simulink model "motor_error"  (R2018b)
settings: Solver=FixedStepAuto  StartTime=0.0  StopTime=10.0  FixedStep=0.001  RelTol=1e-3
settings Model: Creator=chengqian  LastModifiedBy=chengqian

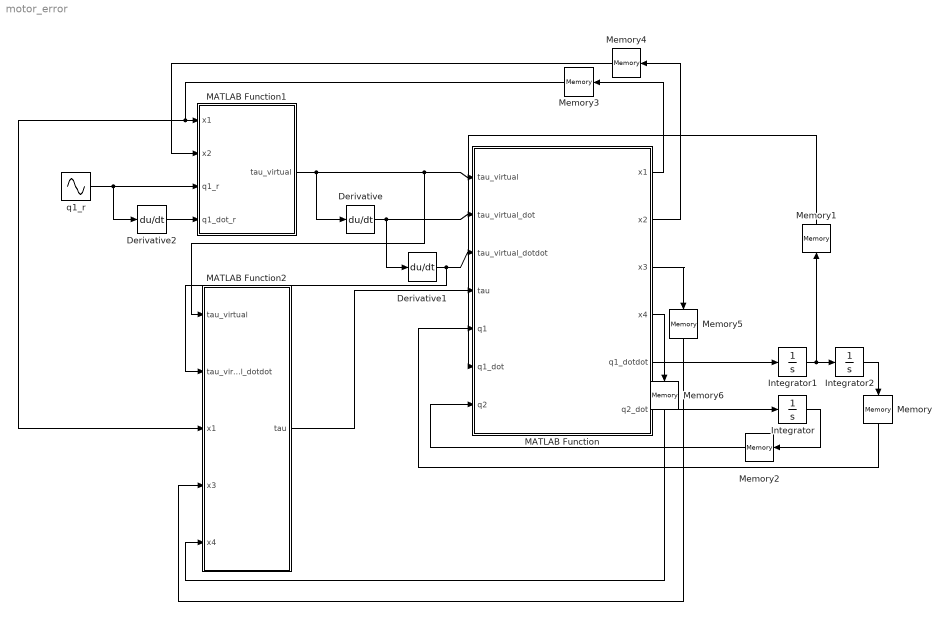
== system motor_error ==
  Derivative : Derivative
  Derivative1 : Derivative
  Derivative2 : Derivative
  Integrator : Integrator
  Integrator1 : Integrator
  Integrator2 : Integrator
  MATLAB Function : MATLAB Function  TreatAsAtomicUnit=on
  MATLAB Function1 : MATLAB Function  TreatAsAtomicUnit=on
  MATLAB Function2 : MATLAB Function  TreatAsAtomicUnit=on
  Memory{,1..6} (7 alike) : Memory
  q1_r : Sin  SampleTime=0
  wires:
  MATLAB Function1/1(tau_virtual) -> Derivative/1, MATLAB Function2/1(tau_virtual), MATLAB Function/1(tau_virtual)
  Derivative/1 -> Derivative1/1, MATLAB Function/2(tau_virtual_dot)
  Derivative1/1 -> MATLAB Function2/2(tau_virtual_dotdot), MATLAB Function/3(tau_virtual_dotdot)
  MATLAB Function/6(q2_dot) -> Integrator/1
  Integrator/1 -> Memory2/1
  MATLAB Function/5(q1_dotdot) -> Integrator1/1
  Integrator2/1 -> Memory/1
  MATLAB Function/1(x1) -> Memory3/1
  MATLAB Function/2(x2) -> Memory4/1
  q1_r/1 -> Derivative2/1, MATLAB Function1/3(q1_r)
  Derivative2/1 -> MATLAB Function1/4(q1_dot_r)
  MATLAB Function2/1(tau) -> MATLAB Function/4(tau)
  MATLAB Function/4(x4) -> Memory6/1
  MATLAB Function/3(x3) -> Memory5/1
  Integrator1/1 -> Integrator2/1, Memory1/1
  Memory/1 -> MATLAB Function/5(q1)
  Memory1/1 -> MATLAB Function/6(q1_dot)
  Memory2/1 -> MATLAB Function/7(q2)
  Memory3/1 -> MATLAB Function2/3(x1), MATLAB Function1/1(x1)
  Memory4/1 -> MATLAB Function1/2(x2)
  Memory5/1 -> MATLAB Function2/4(x3)
  Memory6/1 -> MATLAB Function2/5(x4)

== matlab function motor_error/MATLAB Function1 ==
  data: x1 input; tau_virtual output; x2 input; q1_r input; q1_dot_r input
function tau_virtual = fcn(x1,x2,q1_r,q1_dot_r)

T = 10;
J = 0.0101;
M = 0.0320;
K = 4000;

beta1 = 2; beta2 = 2;
alpha1 = 10; alpha2 = 10;
Kp1 = 100; Kd1 =20;

rol1 = norm((-T - K*x1 + M*x2));
e1 = q1_r - x1;
e2 = q1_dot_r - x2;
tau_virtual = (1/K)*((-alpha1*rol1^2-beta1)*(x1+x2) + (-Kp1*e1-Kd1*e2));

== matlab function motor_error/MATLAB Function ==
  data: tau_virtual input; tau_virtual_dot input; tau_virtual_dotdot input; tau input; q1 input; q1_dot input; x1 output size=1; q2 input; x2 output size=1; x3 output size=1; x4 output size=1; q1_dotdot output size=1; q2_dot output size=1
function [x1,x2,x3,x4,q1_dotdot,q2_dot] = fcn(tau_virtual,tau_virtual_dot,tau_virtual_dotdot,tau,q1,q1_dot,q2)

T = 10;
J = 0.0101;
M = 0.0320;
K = 4000;

beta1 = 2; beta2 = 2;
alpha1 = 10; alpha2 = 10;
Kp1 = 100; Kd1 =20;

x1 = q1;
x2 = q1_dot;
x3 = q2 - tau_virtual;



q1_dotdot = (- T - K*x1 + K*x3 + K*tau_virtual)/M;
q2_dot = (-J*tau_virtual_dotdot + K*x1 - K*x3 - K*tau_virtual + tau)/J + tau_virtual_dot; 
x4 = q2_dot - tau_virtual_dot;

== matlab function motor_error/MATLAB Function2 ==
  data: tau_virtual input; tau_virtual_dotdot input; x1 input; x3 input; x4 input; tau output
function tau = fcn(tau_virtual,tau_virtual_dotdot,x1,x3,x4)
T = 10;
J = 0.0101;
M = 0.0320;
K = 4000;

beta1 = 2; beta2 = 2;
alpha1 = 10; alpha2 = 10;
Kp1 = 100; Kd1 =20;

rol2 = norm((-J*tau_virtual_dotdot - K*x3 + K*x1 - K*tau_virtual + J*x4));
%e2 = q2_r - x2;
tau = (-alpha2*rol2^2- beta2)*(x4 + x3);
